simulink model "regler_wg_img"  (R2012b)
settings: Solver=ode45  StartTime=0.0  StopTime=10.0  RelTol=1e-3
values from neighbouring files (symbols this model uses):
  dP_thrREF = 10e3    (= 10000)    [Init_Project2.m]
  KpWg = 1e-6    (= 1e-06)    [Init_Project2.m]
  TiWg = 4    [Init_Project2.m]
settings Model: Creator=rasme879  LastModifiedBy=rasme879

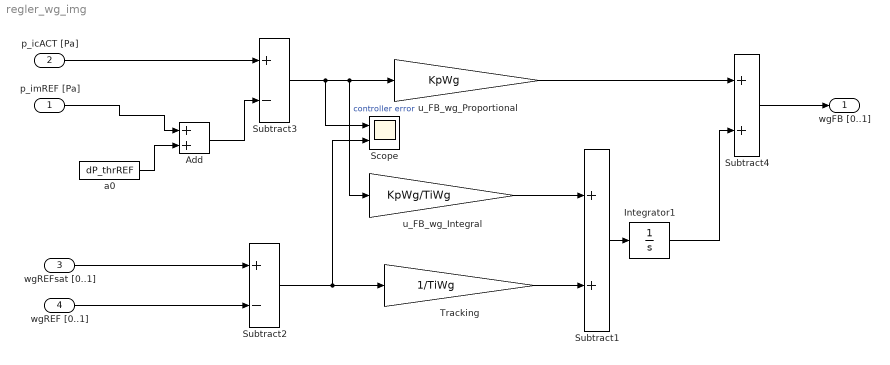
== system regler_wg_img ==
  p_imREF [Pa] : Inport
  p_icACT [Pa] : Inport  Port=2
  wgREFsat [0..1] : Inport  Port=3
  wgREF [0..1] : Inport  Port=4
  Add : Sum
  Integrator1 : Integrator  InitialCondition=1
  Scope : Scope  NumInputPorts=2
      settings: ShowLegends=on  YMin=-50000~-0.085  YMax=100000~0
  Subtract1 : Sum
  Subtract2 : Sum  Inputs=+-
  Subtract3 : Sum  Inputs=+-
  Subtract4 : Sum
  Tracking : Gain  Gain=1/TiWg
  a0 : Constant  Value=dP_thrREF
  u_FB_wg_Integral : Gain  Gain=KpWg/TiWg
  u_FB_wg_Proportional : Gain  Gain=KpWg
  wgFB [0..1] : Outport
  wires:
  Integrator1/1 -> Subtract4/2
  Subtract1/1 -> Integrator1/1
  Tracking/1 -> Subtract1/2
  Subtract2/1 -> Scope/2, Tracking/1
  wgREF [0..1]/1 -> Subtract2/2
  wgREFsat [0..1]/1 -> Subtract2/1
  u_FB_wg_Integral/1 -> Subtract1/1
  Subtract4/1 -> wgFB [0..1]/1
  u_FB_wg_Proportional/1 -> Subtract4/1
  Subtract3/1 -> Scope/1, u_FB_wg_Proportional/1, u_FB_wg_Integral/1  "controller error"
  p_icACT [Pa]/1 -> Subtract3/1
  Add/1 -> Subtract3/2
  a0/1 -> Add/2
  p_imREF [Pa]/1 -> Add/1
